simulink model "demo_microgrid_op4510_2_sc_gui"  (R2017b)
settings: Solver=ode4  StartTime=0.0  StopTime=inf  FixedStep=2e-05  RelTol=1e-3
values from neighbouring files (symbols this model uses):
  DS001_f0 = 50    [Script_Initialization.m]
  DS001_p0 = 500    [Script_Initialization.m]
  f0_vsi_2 = 50    [Script_Initialization.m]
  kp_vsi_2 = (f0_vsi_2/pmax_vsi_2)*3/1000    (= 7.5e-05)    [Script_Initialization.m]
  on_vsi_2 = 1    [Script_Initialization.m]
  p0_vsi_2 = 500    [Script_Initialization.m]
  phi0Deg_vsi_2 = phi0_vsi_2*180/pi    (= 45)    [Script_Initialization.m]
  q0_vsi_2 = 0    [Script_Initialization.m]
  tp_vsi_2 = 100e-3    (= 0.1)    [Script_Initialization.m]
  v0_vsi_2 = 340*sqrt(2)    [Script_Initialization.m]
libraries: opal_lib x2, xpcrtudplib x2, etargetslib x1, embdlinuxlib x1
settings Model: xpc_rtwmakecfg_data=_xpcnblib__xpcetherlib__xpcether8255xlib__xpcetherGbElib__xpciplib_  Creator=Edwin_Mora  LastModifiedBy=EINS_Admin
settings DebuggingCC: UnconnectedInputMsg=none  UnconnectedOutputMsg=none  UnconnectedLineMsg=none
settings RTWCC: GenCodeOnly=on
settings ConfigComp: PSAutoStubLUT=on

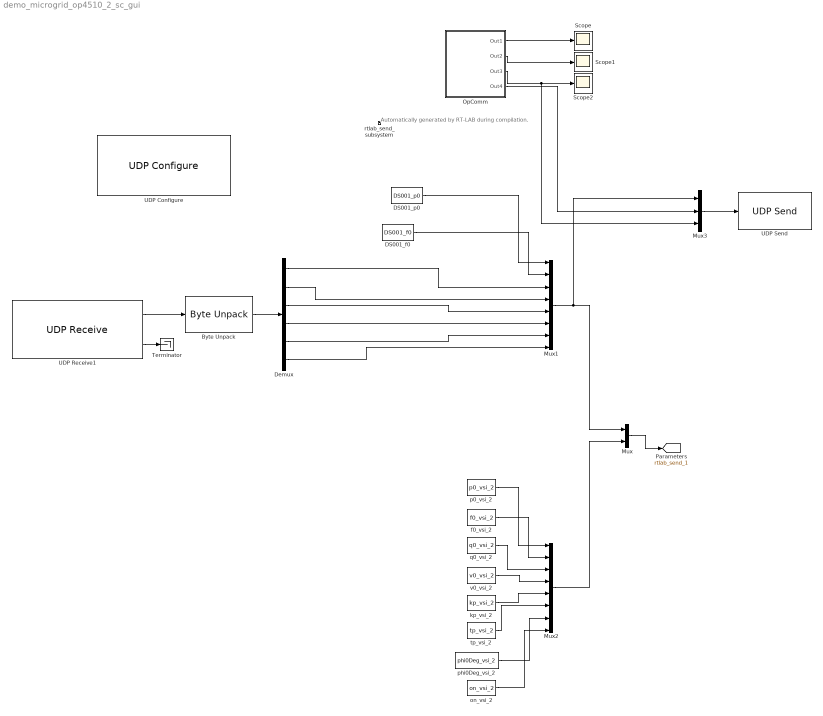
== system demo_microgrid_op4510_2_sc_gui ==
  note: Automatically generated by RT-LAB during compilation.
  Byte Unpack : etargetslib/Byte Unpack  dimensions={[6]}  datatypes={'double'}  byteAlign=1
  DS001_f0 : Constant  Value=DS001_f0
  DS001_p0 : Constant  Value=DS001_p0
  Demux : Demux  Outputs=6
  Mux : Mux  Inputs=2
  Mux1 : Mux  Inputs=8
  Mux2 : Mux  Inputs=8
  Mux3 : Mux  Inputs=3
  OpComm : Subsystem
      mask init:
      | opmaskdisplay('maskdisplay_block',gcb,'disp(''OpComm'')');
      mask Display:
      | patch([0 0.5 0.7 0],[1 1 0 0],[0.7 0.75 0.9]);
      | patch([1 0.53 0.73 1],[1 1 0 0],[1 0.8 0.7]);
      | plot([0 0 1 1 0],[0 1 1 0 0]);
      | disp('OpComm')
  Scope : Scope
  Scope1 : Scope
  Scope2 : Scope
  Terminator : Terminator
  UDP Configure : xpcrtudplib/UDP Configure  Priority=-1  IpAddress=192.168.1.100  SubnetMask=255.255.255.0  Gateway=0.0.0.0  PciBus=[0]  PciSlot=[6]  PciFunction=0  ID=1  tune=0
      settings: SourceProductName=Simulink Real-Time  SourceProductBaseCode=XP
  UDP Receive1 : xpcrtudplib/UDP Receive  ipAddressVal=192.168.1.100  localPort=8002  rcvWidth=48  rcvFmAny=on  fmAddress=0.0.0.0  maxUDPQueue=8  sampleTime=-1
      settings: SourceProductName=Simulink Real-Time
  UDP Send : embdlinuxlib/UDP Send  remoteURL='192.168.1.11'  remotePort=8001  localURL='255.255.255.255'  localPortSource=Automatically determine  localPort=-1  sampletime=-1  blockPlatform=Raspberry Pi  separateLengthPort=0
      settings: SourceProductName=Simulink Support Package for Raspberry Pi Hardware  SourceProductBaseCode=RASPPI
  f0_vsi_2 : Constant  Value=f0_vsi_2
  kp_vsi_2 : Constant  Value=kp_vsi_2
  on_vsi_2 : Constant  Value=on_vsi_2
  p0_vsi_2 : Constant  Value=p0_vsi_2
  phi0Deg_vsi_2 : Constant  Value=phi0Deg_vsi_2
  q0_vsi_2 : Constant  Value=q0_vsi_2
  rtlab_send_subsystem : Subsystem  Priority=-100
      mask Display: text(0,0,'');
  tp_vsi_2 : Constant  Value=tp_vsi_2
  v0_vsi_2 : Constant  Value=v0_vsi_2
  tag scope: rtlab_send_1=global
  wires:
  UDP Receive1/2 -> Terminator/1
  Byte Unpack/1 -> Demux/1
  Demux/6 -> Mux1/8
  Demux/5 -> Mux1/7
  Demux/4 -> Mux1/6
  Demux/3 -> Mux1/5
  Demux/2 -> Mux1/4
  Demux/1 -> Mux1/3
  UDP Receive1/1 -> Byte Unpack/1
  OpComm/4(Out4) -> Mux3/2
  Mux3/1 -> UDP Send/1
  OpComm/2(Out2) -> Scope1/1
  OpComm/3(Out3) -> Mux3/3, Scope2/1
  Mux2/1 -> Mux/2
  v0_vsi_2/1 -> Mux2/4
  phi0Deg_vsi_2/1 -> Mux2/7
  tp_vsi_2/1 -> Mux2/6
  kp_vsi_2/1 -> Mux2/5
  q0_vsi_2/1 -> Mux2/3
  on_vsi_2/1 -> Mux2/8
  p0_vsi_2/1 -> Mux2/1
  f0_vsi_2/1 -> Mux2/2
  Mux1/1 -> Mux3/1, Mux/1
  DS001_f0/1 -> Mux1/2
  DS001_p0/1 -> Mux1/1
  Mux/1 -> [rtlab_send_1]
  OpComm/1(Out1) -> Scope/1

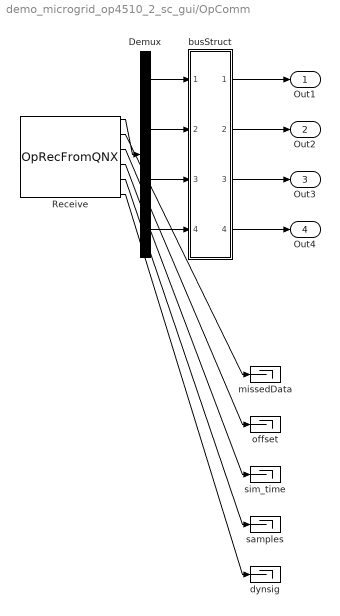
== system demo_microgrid_op4510_2_sc_gui/OpComm ==
  Demux : Demux  Outputs="[1  1  1  1]"
  Receive : opal_lib/Communication/OpRecFromQNX  Node_num=1  Acqu_Group=1  Data_Width=4  Synchronization=on  Interpolation=on  Threshold=1.0  modelname=Demo_Microgrid_OP4510.slx  sampletime=2e-05
  busStruct : Subsystem
  dynsig : Terminator
  missedData : Terminator
  offset : Terminator
  samples : Terminator
  sim_time : Terminator
  Out1 : Outport
  Out2 : Outport  Port=2
  Out3 : Outport  Port=3
  Out4 : Outport  Port=4
  wires:
  Demux/4 -> busStruct/4(In4)
  Demux/3 -> busStruct/3(In3)
  Demux/2 -> busStruct/2(In2)
  Demux/1 -> busStruct/1(In1)
  busStruct/4(Out4) -> Out4/1
  busStruct/3(Out3) -> Out3/1
  busStruct/2(Out2) -> Out2/1
  busStruct/1(Out1) -> Out1/1
  Receive/1 -> Demux/1
  Receive/6 -> dynsig/1
  Receive/5 -> samples/1
  Receive/4 -> sim_time/1
  Receive/3 -> offset/1
  Receive/2 -> missedData/1

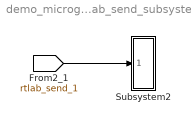
== system demo_microgrid_op4510_2_sc_gui/rtlab_send_subsystem ==
  Subsystem2 : Subsystem
  wires:
  [rtlab_send_1] -> Subsystem2/1(In1)

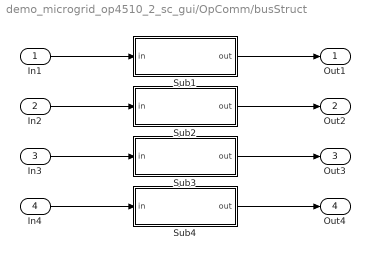
== system demo_microgrid_op4510_2_sc_gui/OpComm/busStruct ==
  In1 : Inport
  In2 : Inport  Port=2
  In3 : Inport  Port=3
  In4 : Inport  Port=4
  Sub1 : Subsystem
  Sub2 : Subsystem
  Sub3 : Subsystem
  Sub4 : Subsystem
  Out1 : Outport
  Out2 : Outport  Port=2
  Out3 : Outport  Port=3
  Out4 : Outport  Port=4
  wires:
  Sub4/1(out) -> Out4/1
  In4/1 -> Sub4/1(in)
  Sub3/1(out) -> Out3/1
  In3/1 -> Sub3/1(in)
  Sub2/1(out) -> Out2/1
  In2/1 -> Sub2/1(in)
  Sub1/1(out) -> Out1/1
  In1/1 -> Sub1/1(in)

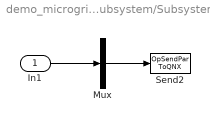
== system demo_microgrid_op4510_2_sc_gui/rtlab_send_subsystem/Subsystem2 ==
  In1 : Inport  PortDimensions=16
  Mux : Mux  Inputs=1
  Send2 : opal_lib/Communication/OpSendPar ToQNX  Node_num=1  modelname=Demo_Microgrid_OP4510
  wires:
  Mux/1 -> Send2/1
  In1/1 -> Mux/1

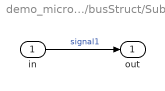
== system demo_microgrid_op4510_2_sc_gui/OpComm/busStruct/Sub1 ==
  in : Inport
  out : Outport
  wires:
  in/1 -> out/1  "signal1"

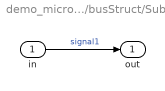
== system demo_microgrid_op4510_2_sc_gui/OpComm/busStruct/Sub2 ==
  in : Inport
  out : Outport
  wires:
  in/1 -> out/1  "signal1"

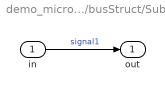
== system demo_microgrid_op4510_2_sc_gui/OpComm/busStruct/Sub3 ==
  in : Inport
  out : Outport
  wires:
  in/1 -> out/1  "signal1"

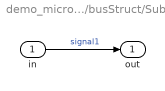
== system demo_microgrid_op4510_2_sc_gui/OpComm/busStruct/Sub4 ==
  in : Inport
  out : Outport
  wires:
  in/1 -> out/1  "signal1"
